simulink model "tmp_old"  (R2018b)
settings: Solver=VariableStepAuto  StartTime=0.0  StopTime=10.0  RelTol=1e-3
undefined symbols (not defined in the file or in its folder): GeRa, sigbuilder_block
libraries: fl_lib x63, sdl_lib x20, nesl_utility x11, simulink x7, dspswit3 x1
(part 1 of 3)
settings Model: Creator=Tanya  LastModifiedBy=Tanya

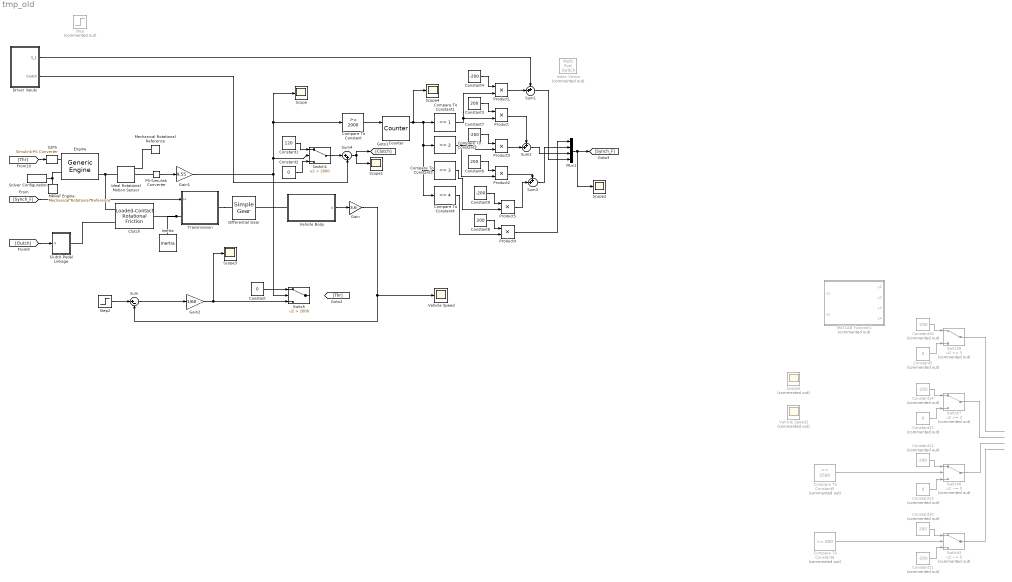
== system tmp_old ==
  Clutch : sdl_lib/Brakes & Detents/Rotational/Loaded-Contact Rotational Friction  geometry_model=1  r_eff=300 mm  d_o=150 mm  d_i=100 mm  friction_model=1  mu_coulomb=0.46  mu_w_vector=[ 0 0.1 0.2 0.3 0.4 0.5 1 2 5 10 100 1000 ] rad/s  mu_coulomb_vector=[ 0.29 0.28 0.26 0.22 0.21 0.2 0.2 0.19 0.19 0.19 0.19 0.19 ]  mu_interp_method=1  mu_extrap_method=1  mu_static=0.5  w_tol=0.001 rad/s  force_min=10 N  mu_visc=0 N*m/(rad/s)  initial_state_locked=0  temperature_TLU=[280.0, 300.0, 320.0] K  mu_coulomb_temp_vector=[0.3, 0.28, 0.25]  mu_coulomb_matrix=[0.34, 0.32, 0.3; 0.3, 0.28, 0.25; 0.25, 0.2, 0.15]  mu_static_vector=[0.4, 0.38, 0.36]  thermal_mass=50 kJ/K  T_init=300 K
      settings: SourceProductName=Simscape Driveline  SourceProductBaseCode=LD
  Clutch Pedal Linkage : Subsystem  Tag=PublishSubsystem
      mask Display:
      | color('white')
      | plot(-40,-80);
      | plot(40,40);
      | color('black'),
      | patch([-45 -30 -20 -20 -45],[-90 -90 -75 -55 -90]+20)
      | patch([-30 -10  5 10 20 [20 10 6 -10 -30]-2],[-55 -50 20 25 35 fliplr([-55 -50 20 25 35])-5]);
  Compare To Constant : simulink/Logic and Bit Operations/Compare To Constant  relop=>=  const=2000  OutDataTypeStr=boolean
  Compare To Constant1 : simulink/Logic and Bit Operations/Compare To Constant  relop===  const=1  OutDataTypeStr=uint8
  Compare To Constant2 : simulink/Logic and Bit Operations/Compare To Constant  relop===  const=2  OutDataTypeStr=uint8
  Compare To Constant3 : simulink/Logic and Bit Operations/Compare To Constant  relop===  const=3  OutDataTypeStr=uint8
  Compare To Constant4 : simulink/Logic and Bit Operations/Compare To Constant  relop===  const=4  OutDataTypeStr=uint8
  Compare To Constant5 : simulink/Logic and Bit Operations/Compare To Constant  Commented=on  relop=>=  const=2500  OutDataTypeStr=uint8
  Compare To Constant6 : simulink/Logic and Bit Operations/Compare To Constant  Commented=on  relop=>=  const=800  OutDataTypeStr=uint8
  Constant : Constant  Value=0
  Constant1 : Constant  Value=120
  Constant10 : Constant  Commented=on  Value=200
  Constant11 : Constant  Commented=on  Value=-200
  Constant12 : Constant  Commented=on  Value=200
  Constant13 : Constant  Commented=on  Value=0
  Constant14 : Constant  Commented=on  Value=-200
  Constant15 : Constant  Commented=on  Value=0
  Constant16 : Constant  Commented=on  Value=-200
  Constant2 : Constant  Value=0
  Constant3 : Constant  Value=200
  Constant4 : Constant  Value=-200
  Constant5 : Constant  Commented=on  Value=0
  Constant6 : Constant  Value=200
  Constant7 : Constant  Value=-200
  Constant8 : Constant  Value=200
  Constant9 : Constant  Value=-200
  Counter : dspswit3/Counter  Direction=Up  CountEvent=Rising edge  CounterSize=User defined  MaxCount=255  InitialCount=0  Output=Count and Hit  HitValue=32  ResetInput=on  SamplesPerFrame=1  Ts=1  CntDtype=double  HitDtype=Logical
  Differential Gear : sdl_lib/Gears/Simple Gear  ratio=4.3  rotation_direction=1  friction_model=2  T_noload=0.1 N*m  T_nom=5 N*m  efficiency_nom=0.8  efficiency=0.86  mu_visc=[0 0] N*m/(rad/s)  w_thr=0.01 rad/s  pwr_thr=0.001 W  enable_faults=0  efficiency_fault=0.05  external_fault=simscape.enum.onoff.off  temporal_fault=0  fault_time=5 s  fault_angles=pi / 12 rad  report_fault=1  temperature_TLU=[ 280 300 320 ] K  load_TLU=[ 1 5 10 ] N*m  efficiency_TLU=[ 0.95 0.9 0.85 ]  efficiency_TLU2=[ 0.85 0.8 0.75; 0.95 0.9 0.85; 0.85 0.8 0.7 ]  thermal_mass=50 J/K  T_init=300 K
      settings: SourceProductName=Simscape Driveline
  Driver inputs : Subsystem  Tag=STV Subsys  LoadFcn=sigbuilder_block('load');  StartFcn=sigbuilder_block('start');  StopFcn=sigbuilder_block('stop');  ClipboardFcn=sigbuilder_block('clipboard');  mask(Sigbuilder block){tuvar=[0:10]}
      mask help: Sigbuilder GUI
      mask init:
      | if ~strcmp(get_param(bdroot(gcbh),'SimulationStatus'),'stopped') tuvar = sigbuilder_block('maskInit'); end
      settings: CopyFcn=sigbuilder_block('copy');  DeleteFcn=sigbuilder_block('delete');  ModelCloseFcn=sigbuilder_block('modelClose');  PreSaveFcn=sigbuilder_block('preSave');  PauseFcn=sigbuilder_block('pause')  ContinueFcn=sigbuilder_block('continue')  NameChangeFcn=sigbuilder_block('namechange');  OpenFcn=sigbuilder_block('open',[187.8 152.4 619.2 435 ]);  CloseFcn=sigbuilder_block('close');
      mask Display: plot(0, 0, 100, 100,[2, 2, 32, 32, 2], [68, 8, 8, 68, 68],[32, 2], [38, 38], [32, 19, 2],[53, 60, 44], [32, 17, 17, 2],[16, 16, 31, 31]);txt = getActiveGroup(gcbh);text(2, 100, txt,'verticalAlignment', 'top');
  Engine : sdl_lib/Engines/Generic Engine  model_parameterization=1  engine_type=1  P_max=100e3 W  w_P_max=6500 rpm  w_max=8500 rpm  w_min=200 rpm  w_tab=[ 500 1000 2e+3 3e+3 4e+3 5e+3 6e+3 7e+3 ] rpm  trq_tab=[ 380 380 380 380 350 280 200 80 ] N*m  pwr_tab=[ 2e+4 4e+4 7.8e+4 1.2e+5 1.45e+5 1.48e+5 1.25e+5 6e+4 ] W  interp_method=simscape.enum.interpolation.linear  model_inertia=1  inertia=0.16 kg*m^2  initial_velocity=800 rpm  model_time_constant=1  time_constant=0.2 s  T0=0  w_thr=20 rpm  idle_speed=1  idle_speed_reference=800 rpm  tau_controller=.6 s  idle_w_thr=1 rpm  redline=0  redline_speed=5000 rpm  tau_redline=1 s  redline_w_thr=1 rpm  fc_model=0  fc_per_rev=25 mg/rev  displaced_volume=400 cm^3  rev_per_cycle=2  fc_w_tab=[ 1000 2e+3 3e+3 4e+3 5e+3 6e+3 ] rpm  fc_trq_tab=[ 0 80 160 200 240 320 360 400 ] N*m  fc_tab=[ 0.5 0.9 1.4 1.6 1.9 2.7 3.4 4.4; 1 1.7 2.7 3.1 3.6 5 6 7.4; 1.4 2.7 4 4.8 5.6 7.5 8.5 10.5; 2 3.6 5.8 6.7 8 10.4 11.7 13.3; 2.5 4.8 7.9 9.4 10.8 14 16.2 18.6; 3.1 6 10.3 11.9 13.8 18.4 22 26.5 ] g/s  bmep_tab=[ 0 250 500 625 750 1000 1.15e+3 1.25e+3 ] kPa  bsfc_tab=[ 410 380 300 280 270 290 320 380; 410 370 290 270 260 270 285 320; 415 380 290 275 265 270 270 300; 420 390 310 290 285 280 280 285; 430 410 340 320 310 300 310 320; 450 430 370 340 330 330 350 380 ] g/hr/kW  fc_interp_method=simscape.enum.interpolation.linear
      settings: SourceProductName=Simscape Driveline  SourceProductBaseCode=LD
  Gain : Gain  Gain=3.6
  Gain1 : Gain  Gain=9.55
  Gain2 : Gain  Gain=1/60
  Ideal Rotational Motion Sensor : fl_lib/Mechanical/Mechanical Sensors/Ideal Rotational Motion Sensor  offset=0 rad
  Index Vector : MultiPortSwitch  Commented=on  DataPortOrder=Zero-based contiguous  Inputs=2  zeroidx=on
  Inertia : fl_lib/Mechanical/Rotational Elements/Inertia  inertia=0.005 kg*m^2  w_specify=off  w_priority=High  w=0 rad/s  w_nominal_specify=off  w_nominal_unit=rad/s  w_nominal_value=1  t_specify=off  t_priority=High  t=0 N*m  t_nominal_specify=off  t_nominal_unit=N*m  t_nominal_value=1
  MATLAB Function1 : MATLAB Function  Commented=on  TreatAsAtomicUnit=on
  MRRef Engine : fl_lib/Mechanical/Rotational Elements/Mechanical Rotational Reference
  Mechanical Rotational Reference : fl_lib/Mechanical/Rotational Elements/Mechanical Rotational Reference
  Mux1 : Mux
  PS-Simulink Converter : nesl_utility/PS-Simulink Converter  PhysicalDomain=network_engine_domain  SubClassName=ps_output  LeftPortType=input  RightPortType=output  PseudoPeriodic=off  Frequencies=[]  Unit=rad/s  AffineConversion=off
  Product{,1..5} (6 alike) : Product
  S2PS : nesl_utility/Simulink-PS Converter  PhysicalDomain=network_engine_domain  SubClassName=ps_input  LeftPortType=input  RightPortType=output  PseudoPeriodic=off  Frequencies=[]  NoiseDistribution=none  NoiseParameters=[]  Unit=1  AffineConversion=off  FilteringAndDerivatives=zero  SimscapeFilterOrder=1  InputFilterTimeConstant=.001  UdotUserProvided=0
  Scope{,1..4} (5 alike) : Scope
  Scope5 : Scope  Commented=on
  Solver Configuration : nesl_utility/Solver Configuration  PhysicalDomain=network_engine_domain  SubClassName=solver  LeftPortType=input  RightPortType=generic  Tones=[]  Harmonics=[]  SimulateNoise=off  Profile=off  UseLocalSampling=off  EnableSwitchedLinearOptims=on  FrequencyDomain=off  UseCCode=off  RelTol=0.001  AbsTol=1e-06  MinStep=1e-09  ToWorkspace=off  RevertToSquareIcSolve=off  NumHomotopyIterations=100  PhasorMode=off  PhasorModeNumHarmonics=1  DoDC=off  ResidualTolerance=1e-9  UseLocalSolver=off  LocalSolverChoice=NE_BACKWARD_EULER_ADVANCER  LocalSolverSampleTime=.001  DoFixedCost=off  MaxNonlinIter=3  MaxModeIter=2  LinearAlgebra=auto  EquationFormulation=NE_TIME_EF  DelaysMemoryBudget=1024  AutomaticFiltering=on  FilteringTimeConstant=0.001  PartitionStorageMethod=AS_NEEDED  PartitionMemoryBudget=1024
  Step : Step  Commented=on  Time=3.6  After=0.1  SampleTime=0
  Step2 : Step  Time=3.6  After=60  SampleTime=0
  Sum : Sum  Inputs=|+-
  Sum1 : Sum  Inputs=++|
  Sum2 : Sum  Inputs=++|
  Sum3 : Sum  Inputs=++|
  Sum4 : Sum  Inputs=|++
  Switch : Switch  Criteria=u2 > Threshold  Threshold=2000
  Switch1 : Switch  Criteria=u2 > Threshold  Threshold=2000
  Switch2 : Switch  Commented=on  Criteria=u2 ~= 0  Threshold=2000
  Switch6 : Switch  Commented=on  Criteria=u2 ~= 0  Threshold=1.6
  Switch7 : Switch  Commented=on  Threshold=2
  Switch8 : Switch  Commented=on  Threshold=3
  Transmission : Subsystem  VariantControlMode=Label  Variant=on  LabelModeActiveChoice=Detailed
      settings: AttributesFormatString=%<ActiveVariant>
      mask Display:
      | blk = find_system(gcbh, 'SearchDepth', 1, 'Parent', gcb, 'VariantObject', get_param(gcb,'activevariant'));
      | eval(get_param(blk, 'MaskDisplay'));
  Vehicle Speed : Scope
  Vehicle Speed1 : Scope  Commented=on
  Vehicle Body : Subsystem  Tag=PublishSubsystem
      mask Display:
      | color('white')
      | plot(-120,-60); plot(120,50);
      | color('black')
      | plot(sin(0:0.1:6*pi)*15-70,cos(0:0.1:6*pi)*15-30);
      | plot(sin(0:0.1:6*pi)*15+70,cos(0:0.1:6*pi)*15-30);
      | plot([-88 -95 -99 -99 -95 -75 -65 -50 -46 10 30 34 80 85 90 93 95 93 90 88],[-30 -28 -23 -5 0 5 10 20 21 21 0 -2 -7 -9 -13 -17 -25 -28 -30 -30])
      | plot([-88 -95 -99 -99 -95 -75 -65 -50 -46 10 30 34 80 85 90 93 95 93 90 88],[-30 -28 -23 -5 0 5 10 20 21 21 0 -2 -7 -9 -13 -17 -25 -28 -30 -30]-1)
      | plot([-88 -95 -99 -99 -95 -75 -65 -50 -46 10 30 34 80 85 90 93 95 93 90 88]+1,[-30 -28 -23 -5 0 5 10 20 21 21 0 -2 -7 -9 -13 -17 -25 -28 -30 -30])
      | plot([-50 50],[-30 -30])
  wires:
  Driver inputs/1(S_1) -> Sum1/1
  Constant6/1 -> Product2/1
  Product2/1 -> Sum3/1
  Constant4/1 -> Product1/1
  Product3/1 -> Sum2/2
  Counter/1 -> Scope4/1, Compare To Constant4/1, Compare To Constant3/1, Compare To Constant2/1, Compare To Constant1/1
  Compare To Constant3/1 -> Product5/2
  Product5/1 -> Sum3/2
  [Clutch] -> Clutch Pedal Linkage/1(S)
  Step2/1 -> Sum/1
  [Synch_F] -> Transmission/1(H)
  Compare To Constant/1 -> Counter/1
  Constant7/1 -> Product3/1
  Product4/1 -> Mux1/1
  Compare To Constant4/1 -> Product4/2
  Vehicle Body/1(V) -> Gain/1
  Constant8/1 -> Product4/1
  Constant9/1 -> Product5/1
  Compare To Constant1/1 -> Product1/2, Product/2
  Product/1 -> Sum2/1
  Mux1/1 -> [Synch_F], Scope2/1
  Constant2/1 -> Switch1/3
  PS-Simulink Converter/1 -> Gain1/1
  Gain2/1 -> Scope3/1, Switch/3
  Sum2/1 -> Mux1/3
  Sum4/1 -> [Clutch], Scope1/1
  Product1/1 -> Sum1/2
  Sum3/1 -> Mux1/2
  Compare To Constant2/1 -> Product2/2, Product3/2
  Constant/1 -> Switch/1
  Switch1/1 -> Sum4/1
  Sum/1 -> Gain2/1
  Constant3/1 -> Product/1
  Driver inputs/2(Clutch) -> Sum4/2
  [Thr] -> S2PS/1
  Sum1/1 -> Mux1/4
  Constant1/1 -> Switch1/1
  Gain1/1 -> Scope/1, Compare To Constant/1, Switch1/2, Switch/2
  Gain/1 -> Sum/2, Vehicle Speed/1
  Switch7/1 -> ?
  ? -> MATLAB Function1/1(u1), Switch8/2, Switch7/2, Compare To Constant5/1, Compare To Constant6/1, Scope5/1
  Constant16/1 -> Switch8/1
  Compare To Constant6/1 -> Switch2/2
  Constant5/1 -> Switch8/3
  Switch8/1 -> ?
  Compare To Constant5/1 -> Switch6/2
  Constant10/1 -> Switch2/1
  Constant14/1 -> Switch7/1
  Constant12/1 -> Switch6/1
  Switch6/1 -> ?
  ? -> Vehicle Speed1/1
  Switch2/1 -> ?
  Constant13/1 -> Switch6/3
  Constant11/1 -> Switch2/3
  Constant15/1 -> Switch7/3
  connections:
  MRRef Engine/LConn1 -- Solver Configuration/RConn1 -- Engine/LConn2
  Transmission/LConn1 -- Clutch/RConn1 -- Inertia/LConn1
  Ideal Rotational Motion Sensor/LConn1 -- Clutch/LConn2 -- Engine/RConn3
  Mechanical Rotational Reference/LConn1 -- Ideal Rotational Motion Sensor/RConn1
  Engine/LConn1 -- S2PS/RConn1
  Clutch/LConn1 -- Clutch Pedal Linkage/RConn1
  Transmission/RConn1 -- Differential Gear/LConn1
  PS-Simulink Converter/LConn1 -- Ideal Rotational Motion Sensor/RConn2
  Vehicle Body/LConn1 -- Differential Gear/RConn1

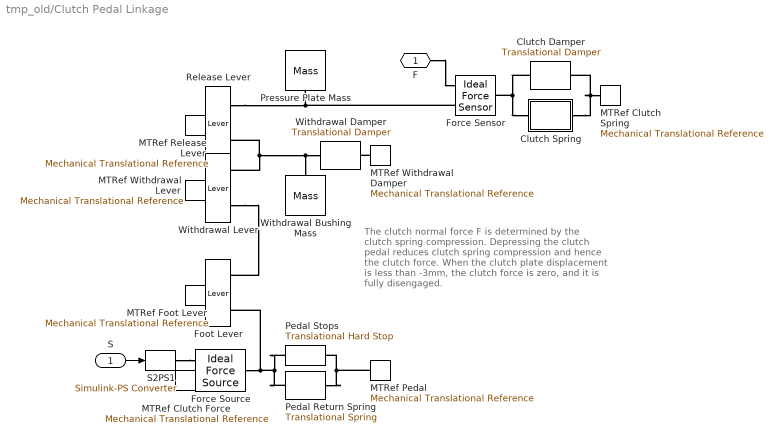
== system tmp_old/Clutch Pedal Linkage ==
  note: The clutch normal force F is determined by the
      | clutch spring compression. Depressing the
      | clutch pedal reduces clutch spring compression
      | and hence the clutch force. When the clutch plate
      | displacement is less than -3mm, the
      | clutch force is zero, and it is fully disengaged.
  S : Inport
  Clutch Damper : fl_lib/Mechanical/Translational Elements/Translational Damper  D=100 N/(m/s)  v_specify=off  v_priority=High  v=0 m/s  v_nominal_specify=off  v_nominal_unit=m/s  v_nominal_value=1  f_specify=off  f_priority=High  f=0 N  f_nominal_specify=off  f_nominal_unit=N  f_nominal_value=1
  Clutch Spring : Subsystem
  Foot Lever : fl_lib/Mechanical/Mechanisms/Lever  arm_AC=76 mm  arm_BC=148 mm  f_A_specify=off  f_A_priority=High  f_A=0 N  f_A_nominal_specify=off  f_A_nominal_unit=N  f_A_nominal_value=1  f_B_specify=off  f_B_priority=High  f_B=0 N  f_B_nominal_specify=off  f_B_nominal_unit=N  f_B_nominal_value=1  f_C_specify=off  f_C_priority=High  f_C=0 N  f_C_nominal_specify=off  f_C_nominal_unit=N  f_C_nominal_value=1
      settings: SourceProductName=Simscape  SourceProductBaseCode=SS
  Force Sensor : fl_lib/Mechanical/Mechanical Sensors/Ideal Force Sensor
  Force Source : fl_lib/Mechanical/Mechanical Sources/Ideal Force Source
  MTRef Clutch Force : fl_lib/Mechanical/Translational Elements/Mechanical Translational Reference
  MTRef Foot Lever : fl_lib/Mechanical/Translational Elements/Mechanical Translational Reference
  MTRef Release Lever : fl_lib/Mechanical/Translational Elements/Mechanical Translational Reference
  MTRef Withdrawal Damper : fl_lib/Mechanical/Translational Elements/Mechanical Translational Reference
  MTRef Withdrawal Lever : fl_lib/Mechanical/Translational Elements/Mechanical Translational Reference
  "MTRef Clutch Spring " : fl_lib/Mechanical/Translational Elements/Mechanical Translational Reference
  MTRef Pedal : fl_lib/Mechanical/Translational Elements/Mechanical Translational Reference
  Pedal Return Spring : fl_lib/Mechanical/Translational Elements/Translational Spring  spr_rate=120 N/m  v_specify=off  v_priority=High  v=0 m/s  v_nominal_specify=off  v_nominal_unit=m/s  v_nominal_value=1  f_specify=off  f_priority=High  f=0 N  f_nominal_specify=off  f_nominal_unit=N  f_nominal_value=1  x_specify=on  x_priority=High  x=1.5 cm  x_nominal_specify=off  x_nominal_unit=m  x_nominal_value=1
  Pedal Stops : fl_lib/Mechanical/Translational Elements/Translational Hard Stop  upper_bnd=168 mm  lower_bnd=0 mm  stiff_up=1e6 N/m  stiff_low=1e6 N/m  D_up=150 N/(m/s)  D_low=150 N/(m/s)  model=3  transition=0.1 mm  v_specify=off  v_priority=High  v=0 m/s  v_nominal_specify=off  v_nominal_unit=m/s  v_nominal_value=1  f_specify=off  f_priority=High  f=0 N  f_nominal_specify=off  f_nominal_unit=N  f_nominal_value=1  x_specify=off  x_priority=High  x=0 m  x_nominal_specify=off  x_nominal_unit=m  x_nominal_value=1
  Pressure Plate Mass : fl_lib/Mechanical/Translational Elements/Mass  mass=4.2 kg  v_specify=off  v_priority=High  v=0 m/s  v_nominal_specify=off  v_nominal_unit=m/s  v_nominal_value=1  f_specify=off  f_priority=High  f=0 N  f_nominal_specify=off  f_nominal_unit=N  f_nominal_value=1
  Release Lever : fl_lib/Mechanical/Mechanisms/Lever  arm_AC=7.2 mm  arm_BC=38 mm  f_A_specify=off  f_A_priority=High  f_A=0 N  f_A_nominal_specify=off  f_A_nominal_unit=N  f_A_nominal_value=1  f_B_specify=off  f_B_priority=High  f_B=0 N  f_B_nominal_specify=off  f_B_nominal_unit=N  f_B_nominal_value=1  f_C_specify=off  f_C_priority=High  f_C=0 N  f_C_nominal_specify=off  f_C_nominal_unit=N  f_C_nominal_value=1
      settings: SourceProductName=Simscape  SourceProductBaseCode=SS
  S2PS1 : nesl_utility/Simulink-PS Converter  PhysicalDomain=network_engine_domain  SubClassName=ps_input  LeftPortType=input  RightPortType=output  PseudoPeriodic=off  Frequencies=[]  NoiseDistribution=none  NoiseParameters=[]  Unit=1  AffineConversion=off  FilteringAndDerivatives=filter  SimscapeFilterOrder=1  InputFilterTimeConstant=.001  UdotUserProvided=0
  Withdrawal Bushing Mass : fl_lib/Mechanical/Translational Elements/Mass  mass=0.6 kg  v_specify=off  v_priority=High  v=0 m/s  v_nominal_specify=off  v_nominal_unit=m/s  v_nominal_value=1  f_specify=off  f_priority=High  f=0 N  f_nominal_specify=off  f_nominal_unit=N  f_nominal_value=1
  Withdrawal Lever : fl_lib/Mechanical/Mechanisms/Lever  arm_AC=42 mm  arm_BC=128 mm  f_A_specify=off  f_A_priority=High  f_A=0 N  f_A_nominal_specify=off  f_A_nominal_unit=N  f_A_nominal_value=1  f_B_specify=off  f_B_priority=High  f_B=0 N  f_B_nominal_specify=off  f_B_nominal_unit=N  f_B_nominal_value=1  f_C_specify=off  f_C_priority=High  f_C=0 N  f_C_nominal_specify=off  f_C_nominal_unit=N  f_C_nominal_value=1
      settings: SourceProductName=Simscape  SourceProductBaseCode=SS
  Withdrawal Damper : fl_lib/Mechanical/Translational Elements/Translational Damper  D=100 N/(m/s)  v_specify=off  v_priority=High  v=0 m/s  v_nominal_specify=off  v_nominal_unit=m/s  v_nominal_value=1  f_specify=off  f_priority=High  f=0 N  f_nominal_specify=off  f_nominal_unit=N  f_nominal_value=1
  F : PMIOPort  Side=Right
  wires:
  S/1 -> S2PS1/1
  connections:
  MTRef Foot Lever/LConn1 -- Foot Lever/RConn1
  MTRef Pedal/LConn1 -- Pedal Return Spring/RConn1 -- Pedal Stops/RConn1
  MTRef Withdrawal Damper/LConn1 -- Withdrawal Damper/RConn1
  MTRef Release Lever/LConn1 -- Release Lever/RConn1
  Withdrawal Lever/LConn2 -- Foot Lever/LConn1
  MTRef Withdrawal Lever/LConn1 -- Withdrawal Lever/RConn1
  Withdrawal Lever/LConn1 -- Release Lever/LConn2 -- Withdrawal Bushing Mass/LConn1 -- Withdrawal Damper/LConn1
  Release Lever/LConn1 -- Force Sensor/RConn1 -- Pressure Plate Mass/LConn1
  Pedal Stops/LConn1 -- Pedal Return Spring/LConn1 -- Force Source/LConn1 -- Foot Lever/LConn2
  "MTRef Clutch Spring "/LConn1 -- Clutch Spring/RConn1 -- Clutch Damper/RConn1
  Clutch Spring/LConn1 -- Clutch Damper/LConn1 -- Force Sensor/LConn1
  F/RConn1 -- Force Sensor/RConn2
  MTRef Clutch Force/LConn1 -- Force Source/RConn2
  S2PS1/RConn1 -- Force Source/RConn1

== system tmp_old/Driver inputs ==
  Demux : Demux  Tag=STV Demux  Outputs=2
  FromWs : FromWorkspace  Tag=STV FromWs  VariableName=tuvar  SampleTime=0
      SigBuilderData=|
      | common.afterFinalStr = 'Extrapolate'
      | common.sampleTime = 0
      | dataSet.timeRange = [0 30]
      | dataSet.name = 'Group 1'
      | sbobj.Groups.Name = 'Group 1'
      | sbobj.Groups.Signals(1).Name = 'S_1'
      | sbobj.Groups.Signals(1).XData = [0 1.7 1.85 3.25 3.35 8.35 8.5 9.3 9.3 9.4 30]
      | sbobj.Groups.Signals(1).YData = [0 0 200 200 0 0 0 -2 0 0 0]
      | sbobj.Groups.Signals(2).Name = 'Clutch'
      | sbobj.Groups.Signals(2).XData = [0 0.95 1.45 3.5 4 8.15 8.35 8.35 10 10.4 15.4 15.8 17.2 17.7 22.5 22.8 24.3 24.6 30]
      | sbobj.Groups.Signals(2).YData = [0 0 120 120 0 0 1 0 0 0 0 0 0 0 0 0 0 0 0]
      | sbobj.Groups.TimeRange = [0 30]
  S_1 : Outport  Tag=STV Outport
  Clutch : Outport  Tag=STV Outport  Port=2
  wires:
  FromWs/1 -> Demux/1
  Demux/1 -> S_1/1
  Demux/2 -> Clutch/1

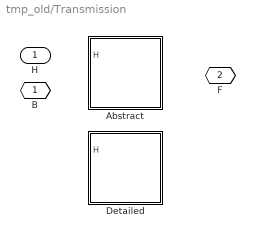
== system tmp_old/Transmission ==
  H : Inport
  Abstract : Subsystem  Tag=PublishSubsystem  VariantControl=Abstract
      mask Display:
      | patch([-20;320.146012604237;320.146012604237;-20;-20], [340.146012604237;340.146012604237;0;0;340.146012604237],[1 1 1])
      | plot([195.583957247436;209.756707772613], [274.951360188425;260.778609663248])
      | plot([209.756707772613;195.583957247436], [274.951360188425;260.778609663248])
      | plot([184.245756827295;198.418507352471], [76.5328528359532;62.3601023107767])
      | plot([198.418507352471;184.245756827295], [76.5328528359532;62.3601023107767])
      | plot([99.2092536762357;99.2092536762357;141.727505251765;141.727505251765;99.2092536762357], [325.97326207906;212.591257877648;255.109509453177;283.455010503531;325.97326207906])
      | patch([136.058405041695;184.245756827295;198.418507352471;121.885654516518;136.058405041695], [289.124110713601;289.124110713601;303.296861238778;303.296861238778;289.124110713601], [0;0;0])
      | plot([136.058405041695;184.245756827295;198.418507352471;121.885654516518;136.058405041695], [289.124110713601;289.124110713601;303.296861238778;303.296861238778;289.124110713601])
      | patch([141.727505251765;141.727505251765;178.576656617224;178.576656617224;141.727505251765], [274.951360188425;266.447709873319;266.447709873319;274.951360188425;274.951360188425], [0;0;0])
      | plot([141.727505251765;141.727505251765;178.576656617224;178.576656617224;141.727505251765], [274.951360188425;266.447709873319;266.447709873319;274.951360188425;274.951360188425])
      | plot([221.094908192754;221.094908192754;178.576656617224;178.576656617224;221.094908192754], [325.97326207906;212.591257877648;255.109509453177;283.455010503531;325.97326207906])
      | patch([70.8637526258826;70.8637526258826;99.2092536762357;99.2092536762357;70.8637526258826], [272.116810083389;263.613159768283;263.613159768283;272.116810083389;272.116810083389], [0;0;0])
      | plot([70.8637526258826;70.8637526258826;99.2092536762357;99.2092536762357;70.8637526258826], [272.116810083389;263.613159768283;263.613159768283;272.116810083389;272.116810083389])
      | patch([221.094908192754;221.094908192754;249.440409243107;249.440409243107;221.094908192754], [272.116810083389;263.613159768283;263.613159768283;272.116810083389;272.116810083389], [0;0;0])
      | plot([221.094908192754;221.094908192754;249.440409243107;249.440409243107;221.094908192754], [272.116810083389;263.613159768283;263.613159768283;272.116810083389;272.116810083389])
      | plot([198.418507352471;198.418507352471], [235.26765871793;119.051104411483])
      | plot([121.885654516518;121.885654516518], [235.26765871793;119.051104411483])
      | plot([113.382004201412;113.382004201412;155.900255776942;155.900255776942;113.382004201412], [127.554754726589;14.1727505251765;56.6910021007061;85.0365031510592;127.554754726589])
      | patch([136.058405041695;184.245756827295;198.418507352471;121.885654516518;136.058405041695], [36.849151365459;36.849151365459;22.6764008402824;22.6764008402824;36.849151365459], [0;0;0])
      | plot([136.058405041695;184.245756827295;198.418507352471;121.885654516518;136.058405041695], [36.849151365459;36.849151365459;22.6764008402824;22.6764008402824;36.849151365459])
      | patch([85.0365031510592;85.0365031510592;113.382004201412;113.382004201412;85.0365031510592], [73.6983027309179;65.194652415812;65.194652415812;73.6983027309179;73.6983027309179], [0;0;0])
      | plot([85.0365031510592;85.0365031510592;113.382004201412;113.382004201412;85.0365031510592], [73.6983027309179;65.194652415812;65.194652415812;73.6983027309179;73.6983027309179])
      | plot([206.922157667577;206.922157667577;164.403906092048;164.403906092048;206.922157667577], [127.554754726589;14.1727505251765;56.6910021007061;85.0365031510592;127.554754726589])
      | patch([206.922157667577;206.922157667577;246.605859138072;246.605859138072;206.922157667577], [73.6983027309179;65.194652415812;65.194652415812;73.6983027309179;73.6983027309179], [0;0;0])
      | plot([206.922157667577;206.922157667577;246.605859138072;246.605859138072;206.922157667577], [73.6983027309179;65.194652415812;65.194652415812;73.6983027309179;73.6983027309179])
      | patch([155.900255776942;155.900255776942;164.403906092048;164.403906092048;155.900255776942], [76.5328528359532;68.0292025208473;68.0292025208473;76.5328528359532;76.5328528359532], [0;0;0])
      | plot([155.900255776942;155.900255776942;164.403906092048;164.403906092048;155.900255776942], [76.5328528359532;68.0292025208473;68.0292025208473;76.5328528359532;76.5328528359532])
  Detailed : Subsystem  Tag=PublishSubsystem  VariantControl=Detailed
      mask Display:
      | plot([225.488460855559;225.439323974897;225.292386547934;225.049063662416;224.711698650743;224.283540522401;223.76871267422;223.172173179813;222.499667040612;221.757670858367;220.953330461928;220.094392089012;219.189127785692;218.246255742078;217.274856331375;216.28428466093;215.284080477431;214.283876293932;213.293304623488;212.321905212785;211.379033169171;210.473768865851;209.614830492935;208.810490096496;208.068493914251;207.39598777505;206.799448280642;206.284620432462;205.85646230412;205.519097292447;205.275774406929;205.128836979966;205.079700099304;205.128836979966;205.275774406929;205.519097292447;205.85646230412;206.284620432462;206.799448280642;207.39598777505;208.068493914251;208.810490096496;209.614830492935;210.473768865851;211.379033169171;212.321905212785;213.293304623488;214.283876293932;215.284080477431;216.28428466093;217.274856331375;218.246255742078;219.189127785692;220.094392089012;220.953330461928;221.757670858367;222.499667040612;223.172173179813;223.76871267422;224.283540522401;224.711698650743;225.049063662416;225.292386547934;225.439323974897;225.488460855559;225.488460855559], [194.182429695502;193.182225512003;192.191653841558;191.220254430856;190.277382387241;189.372118083922;188.513179711005;187.708839314567;186.966843132321;186.29433699312;185.697797498713;185.182969650533;184.75481152219;184.417446510518;184.174123624999;184.027186198036;183.978049317375;184.027186198036;184.174123624999;184.417446510518;184.75481152219;185.182969650533;185.697797498713;186.29433699312;186.966843132321;187.708839314567;188.513179711005;189.372118083922;190.277382387241;191.220254430856;192.191653841558;193.182225512003;194.182429695502;195.182633879001;196.173205549446;197.144604960148;198.087477003763;198.992741307082;199.851679679999;200.656020076437;201.398016258683;202.070522397884;202.667061892291;203.181889740471;203.610047868813;203.947412880486;204.190735766005;204.337673192967;204.386810073629;204.337673192967;204.190735766005;203.947412880486;203.610047868813;203.181889740471;202.667061892291;202.070522397884;201.398016258683;200.656020076437;199.851679679999;198.992741307082;198.087477003763;197.144604960148;196.173205549446;195.182633879001;194.182429695502;194.182429695502])
      | plot([225.488460855559;225.439323974897;225.292386547934;225.049063662416;224.711698650743;224.283540522401;223.76871267422;223.172173179813;222.499667040612;221.757670858367;220.953330461928;220.094392089012;219.189127785692;218.246255742078;217.274856331375;216.28428466093;215.284080477431;214.283876293932;213.293304623488;212.321905212785;211.379033169171;210.473768865851;209.614830492935;208.810490096496;208.068493914251;207.39598777505;206.799448280642;206.284620432462;205.85646230412;205.519097292447;205.275774406929;205.128836979966;205.079700099304;205.128836979966;205.275774406929;205.519097292447;205.85646230412;206.284620432462;206.799448280642;207.39598777505;208.068493914251;208.810490096496;209.614830492935;210.473768865851;211.379033169171;212.321905212785;213.293304623488;214.283876293932;215.284080477431;216.28428466093;217.274856331375;218.246255742078;219.189127785692;220.094392089012;220.953330461928;221.757670858367;222.499667040612;223.172173179813;223.76871267422;224.283540522401;224.711698650743;225.049063662416;225.292386547934;225.439323974897;225.488460855559;225.488460855559], [155.002648243681;154.002444060182;153.011872389737;152.040472979034;151.09760093542;150.1923366321;149.333398259184;148.529057862746;147.7870616805;147.114555541299;146.518016046892;146.003188198711;145.575030070369;145.237665058697;144.994342173178;144.847404746215;144.798267865553;144.847404746215;144.994342173178;145.237665058697;145.575030070369;146.003188198711;146.518016046892;147.114555541299;147.7870616805;148.529057862746;149.333398259184;150.1923366321;151.09760093542;152.040472979034;153.011872389737;154.002444060182;155.002648243681;156.00285242718;156.993424097624;157.964823508327;158.907695551941;159.812959855261;160.671898228177;161.476238624616;162.218234806861;162.890740946062;163.48728044047;164.00210828865;164.430266416992;164.767631428665;165.010954314183;165.157891741146;165.207028621808;165.157891741146;165.010954314183;164.767631428665;164.430266416992;164.00210828865;163.48728044047;162.890740946062;162.218234806861;161.476238624616;160.671898228177;159.812959855261;158.907695551941;157.964823508327;156.993424097625;156.00285242718;155.002648243681;155.002648243681])
      | plot([137.995347613469;137.946210732807;137.799273305844;137.555950420326;137.218585408653;136.790427280311;136.275599432131;135.679059937724;135.006553798522;134.264557616277;133.460217219838;132.601278846922;131.696014543602;130.753142499988;129.781743089286;128.791171418841;127.790967235342;126.790763051843;125.800191381398;124.828791970695;123.885919927081;122.980655623761;122.121717250845;121.317376854407;120.575380672161;119.90287453296;119.306335038553;118.791507190372;118.36334906203;118.025984050358;117.782661164839;117.635723737876;117.586586857215;117.635723737876;117.782661164839;118.025984050358;118.36334906203;118.791507190372;119.306335038553;119.90287453296;120.575380672161;121.317376854407;122.121717250845;122.980655623761;123.885919927081;124.828791970695;125.800191381398;126.790763051843;127.790967235342;128.791171418841;129.781743089286;130.753142499988;131.696014543602;132.601278846922;133.460217219838;134.264557616277;135.006553798522;135.679059937723;136.275599432131;136.790427280311;137.218585408653;137.555950420326;137.799273305844;137.946210732807;137.995347613469;137.995347613469], [275.187572697178;274.187368513678;273.196796843234;272.225397432531;271.282525388917;270.377261085597;269.518322712681;268.713982316242;267.971986133997;267.299479994796;266.702940500388;266.188112652208;265.759954523866;265.422589512193;265.179266626675;265.032329199712;264.98319231905;265.032329199712;265.179266626675;265.422589512193;265.759954523866;266.188112652208;266.702940500389;267.299479994796;267.971986133997;268.713982316242;269.518322712681;270.377261085597;271.282525388917;272.225397432531;273.196796843234;274.187368513678;275.187572697178;276.187776880677;277.178348551121;278.149747961824;279.092620005438;279.997884308758;280.856822681674;281.661163078113;282.403159260358;283.075665399559;283.672204893967;284.187032742147;284.615190870489;284.952555882162;285.19587876768;285.342816194643;285.391953075305;285.342816194643;285.19587876768;284.952555882162;284.615190870489;284.187032742147;283.672204893967;283.075665399559;282.403159260358;281.661163078113;280.856822681674;279.997884308758;279.092620005438;278.149747961824;277.178348551121;276.187776880677;275.187572697178;275.187572697178])
      | plot([99.4454661849886;116.4527668152;116.4527668152;139.129167655483;139.129167655483;198.654719861224;156.136468285695;156.136468285695;195.820169756189;99.4454661849886;99.4454661849886], [272.353022592142;272.353022592142;241.172971436754;241.172971436754;272.353022592142;272.353022592142;229.834771016613;116.4527668152;73.9345152396709;73.9345152396709;272.353022592142])
      | plot([113.618216710165;127.790967235342;141.963717760518;190.151069546118;190.151069546118;161.805568495765;161.805568495765], [278.022122802213;295.029423432425;278.022122802213;278.022122802213;303.533073747531;303.533073747531;278.022122802213])
      | plot([113.618216710165;127.790967235342;141.963717760518;190.151069546118;190.151069546118;161.805568495765;161.805568495765], [68.2654150296003;51.2581143993884;68.2654150296003;68.2654150296003;42.7544640842825;42.7544640842825;68.2654150296003])
      | plot([161.805568495765;190.151069546118], [303.533073747531;278.022122802213])
      | plot([161.805568495765;190.151069546118], [278.022122802213;303.533073747531])
      | plot([161.805568495765;190.151069546118], [68.2654150296003;42.7544640842825])
      | plot([161.805568495765;190.151069546118], [42.7544640842825;68.2654150296003])
      | plot([241.172971436754;278.022122802213], [272.353022592142;272.353022592142])
      | plot([241.172971436754;278.022122802213], [73.9345152396709;73.9345152396709])
      | plot([241.172971436754;278.022122802213], [272.353022592142;303.533073747531])
      | plot([241.172971436754;278.022122802213], [303.533073747531;272.353022592142])
      | plot([241.172971436754;278.022122802213], [73.9345152396709;42.7544640842825])
      | plot([241.172971436754;278.022122802213], [42.7544640842825;73.9345152396709])
      | plot([184.481969336048;227.000220911577;241.172971436754;241.172971436754;278.022122802213;278.022122802213;278.022122802213;241.172971436754;241.172971436754;227.000220911577;184.481969336048;184.481969336048], [229.834771016613;272.353022592142;272.353022592142;303.533073747531;303.533073747531;244.007521541789;42.7544640842825;42.7544640842825;73.9345152396709;73.9345152396709;116.4527668152;229.834771016613])
      | plot([184.481969336048;249.67662175186;249.67662175186;184.481969336048], [215.662020491436;215.662020491436;130.625517340377;130.625517340377])
      | plot([207.15837017633;224.165670806542], [207.15837017633;207.15837017633])
      | plot([207.15837017633;224.165670806542], [141.963717760518;141.963717760518])
      | %plot([71.0999651346356;227.000220911577], [173.143768915907;173.143768915907])
      | plot([136.294617550448;116.4527668152;136.294617550448;119.287316920236;136.294617550448;119.287316920236;136.294617550448;119.287316920236], [269.518472487107;269.518472487107;261.014822172001;258.180272066966;252.511171856895;249.67662175186;246.842071646824;241.172971436754])
      | %plot([0.236212508752942;71.0999651346356;71.0999651346356], [258.180272066966;258.180272066966;278.022122802213])
      | %plot([0.236212508752942;71.0999651346356;71.0999651346356], [88.1072657648474;88.1072657648474;173.143768915907])
      | patch([0;357.625738251954;357.625738251954;0;0;0.472425017505884;0.472425017505884;357.153313234448;357.153313234448;0.472425017505884;0], [343.452987726778;343.452987726778;0;0;343.452987726778;342.980562709272;0.472425017505884;0.472425017505884;342.980562709272;342.980562709272;343.452987726778], [1;1;1])
      | plot([99.4454661849886;113.618216710165], [244.007521541789;258.180272066966])
      | plot([99.4454661849886;124.956417130306], [215.662020491436;241.172971436754])
      | plot([99.4454661849886;184.481969336048], [187.316519441083;272.353022592142])
      | plot([139.129167655483;156.136468285695], [255.34572196193;272.353022592142])
      | plot([99.4454661849886;156.136468285695], [158.97101839073;215.662020491436])
      | plot([99.4454661849886;156.136468285695], [130.625517340377;187.316519441083])
      | plot([99.4454661849886;156.136468285695], [102.280016290024;158.97101839073])
      | plot([99.4454661849886;156.136468285695], [73.9345152396709;130.625517340377])
      | plot([127.790967235342;161.805568495765], [73.9345152396709;110.78366660513])
      | plot([156.136468285695;175.978319020942], [73.9345152396709;93.776365974918])
      | plot([255.34572196193;278.022122802213], [272.353022592142;249.67662175186])
      | plot([227.000220911577;278.022122802213], [272.353022592142;221.331120701507])
      | plot([212.827470386401;278.022122802213], [258.180272066966;192.985619651154])
      | plot([198.654719861224;227.000220911577], [244.007521541789;215.662020491436])
      | plot([249.67662175186;278.022122802213], [192.985619651154;164.640118600801])
      | plot([198.654719861224;184.481969336048], [215.662020491436;229.834771016613])
      | plot([249.67662175186;278.022122802213], [164.640118600801;136.294617550448])
      | plot([249.67662175186;278.022122802213], [139.129167655483;110.78366660513])
      | plot([278.022122802213;227.000220911577], [79.6036154497415;130.625517340377])
      | plot([198.654719861224;255.34572196193], [130.625517340377;73.9345152396709])
  B : PMIOPort  Side=Left
  F : PMIOPort  Port=2  Side=Right

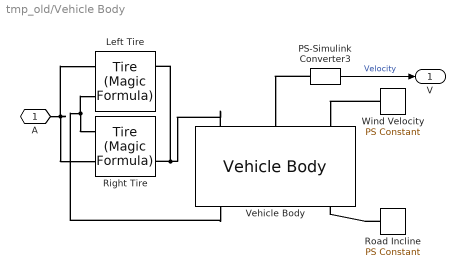
== system tmp_old/Vehicle Body ==
  Left Tire : sdl_lib/Tires & Vehicles/Tire (Magic Formula)  parameterization=3  F_z1=3000 N  F_x1=3500 N  kappa1=10  B_m=10  C_m=1.9  D_m=1  E_m=0.97  fz0=4e+3 N  p_Cx=1.685  p_Dx=[ 1.21 -0.037 ]  p_Ex=[ 0.344 0.095 -0.02 0 ]  p_Kx=[ 21.51 -0.163 0.245 ]  p_Hx=[ -0.002 0.002 ]  p_Vx=[ 0 0 ]  v_tr_thr=0.1 m/s  r_e=0.329 m  model_compliance=0  stiffness=1e+6 N/m  damping=1000 N/(m/s)  model_inertia=1  inertia=0.8 kg*m^2  initial_velocity=0 rpm  model_resistance=0  resistance_model=1  coeff=0.015  p_tire=250e3 Pa  alpha=-0.003  beta=0.97  coeff_a=84e-4  coeff_b=6.2e-4 s/m  coeff_c=1.6e-4 s^2/m^2  v_thr=1e-3 m/s
      settings: SourceProductName=Simscape Driveline
  PS-Simulink Converter3 : nesl_utility/PS-Simulink Converter  PhysicalDomain=network_engine_domain  SubClassName=ps_output  LeftPortType=input  RightPortType=output  PseudoPeriodic=off  Frequencies=[]  Unit=m/s  AffineConversion=off
  Right Tire : sdl_lib/Tires & Vehicles/Tire (Magic Formula)  parameterization=3  F_z1=3000 N  F_x1=3500 N  kappa1=10  B_m=10  C_m=1.9  D_m=1  E_m=0.97  fz0=4e+3 N  p_Cx=1.685  p_Dx=[ 1.21 -0.037 ]  p_Ex=[ 0.344 0.095 -0.02 0 ]  p_Kx=[ 21.51 -0.163 0.245 ]  p_Hx=[ -0.002 0.002 ]  p_Vx=[ 0 0 ]  v_tr_thr=0.1 m/s  r_e=0.329 m  model_compliance=0  stiffness=1e+6 N/m  damping=1000 N/(m/s)  model_inertia=1  inertia=0.8 kg*m^2  initial_velocity=0 rpm  model_resistance=0  resistance_model=1  coeff=0.015  p_tire=250e3 Pa  alpha=-0.003  beta=0.97  coeff_a=84e-4  coeff_b=6.2e-4 s/m  coeff_c=1.6e-4 s^2/m^2  v_thr=1e-3 m/s
      settings: SourceProductName=Simscape Driveline
  Road Incline : fl_lib/Physical Signals/Sources/PS Constant  constant=0
  Vehicle Body : sdl_lib/Tires & Vehicles/Vehicle Body  mass=3500 kg  n_w=2  x_f=1.4 m  x_r=1.6 m  y_c=1 m  model_pitch=0  inertia=4000 kg*m^2  suspension_model=1  k_f=1e4 N/m  b_f=1e4 N/(m/s)  k_r=1e4 N/m  b_r=1e4 N/(m/s)  k_f_TLU=[-2000, -1000, 0, 1000, 2000] N  x_f_TLU=[-.4, -.2, 0, .2, .4] m  b_f_TLU=[-200, -100, 0, 100, 200] N  v_f_TLU=[-4, -2, 0, 2, 4] m/s  k_r_TLU=[-2000, -1000, 0, 1000, 2000] N  x_r_TLU=[-.4, -.2, 0, .2, .4] m  b_r_TLU=[-200, -100, 0, 100, 200] N  v_r_TLU=[-4, -2, 0, 2, 4] m/s  interp_method=simscape.enum.interpolation.linear  extrap_method=simscape.enum.extrapolation.linear  model_hardstop=0  upper_bound_f=.25 m  lower_bound_f=-.25 m  stop_k_f=1e6 N/m  stop_b_f=150 N/(m/s)  upper_bound_r=.25 m  lower_bound_r=-.25 m  stop_k_r=1e6 N/m  stop_b_r=150 N/(m/s)  initial_pitch=0 rad  initial_pitch_rate=0 rad/s  g=9.81 m/s^2  liftoff_warning=0  area=4 m^2  Cd=0.4  rho=1.18 kg/m^3  v_specify=on  v_priority=High  v=0 m/s  v_nominal_specify=off  v_nominal_unit=m/s  v_nominal_value=1
      settings: SourceProductName=Simscape Driveline
  Wind Velocity : fl_lib/Physical Signals/Sources/PS Constant  constant=5
  A : PMIOPort  Side=Left
  V : Outport
  wires:
  PS-Simulink Converter3/1 -> V/1  "Velocity"
  connections:
  Right Tire/RConn2 -- Left Tire/RConn2 -- Vehicle Body/LConn1
  Vehicle Body/RConn1 -- Right Tire/LConn1 -- Left Tire/LConn1
  A/RConn1 -- Right Tire/LConn2 -- Left Tire/LConn2
  PS-Simulink Converter3/LConn1 -- Vehicle Body/LConn2
  Wind Velocity/RConn1 -- Vehicle Body/LConn3
  Road Incline/RConn1 -- Vehicle Body/RConn3

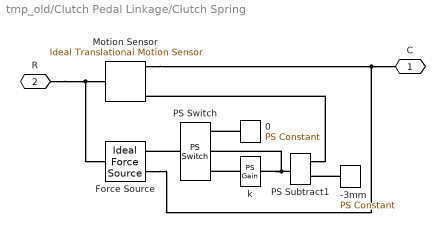
== system tmp_old/Clutch Pedal Linkage/Clutch Spring ==
  -3mm : fl_lib/Physical Signals/Sources/PS Constant  constant=-3e-3
  0 : fl_lib/Physical Signals/Sources/PS Constant  constant=0
  Force Source : fl_lib/Mechanical/Mechanical Sources/Ideal Force Source
  Motion Sensor : fl_lib/Mechanical/Mechanical Sensors/Ideal Translational Motion Sensor  offset=0 m
  PS Subtract1 : fl_lib/Physical Signals/Functions/PS Subtract
      settings: SourceProductName=Simscape
  PS Switch : fl_lib/Physical Signals/Nonlinear Operators/PS Switch  Threshold=0
      settings: SourceProductName=Simscape  SourceProductBaseCode=SS
  k : fl_lib/Physical Signals/Functions/PS Gain  gain=2000/3e-3
  C : PMIOPort  Side=Right
  R : PMIOPort  Port=2  Side=Left
  connections:
  -3mm/RConn1 -- PS Subtract1/LConn2
  Motion Sensor/RConn1 -- Force Source/RConn2 -- C/RConn1
  k/RConn1 -- PS Switch/LConn1
  PS Subtract1/LConn1 -- Motion Sensor/RConn3
  0/RConn1 -- PS Switch/LConn3
  R/RConn1 -- Motion Sensor/LConn1 -- Force Source/LConn1
  PS Subtract1/RConn1 -- PS Switch/LConn2 -- k/LConn1
  PS Switch/RConn1 -- Force Source/RConn1

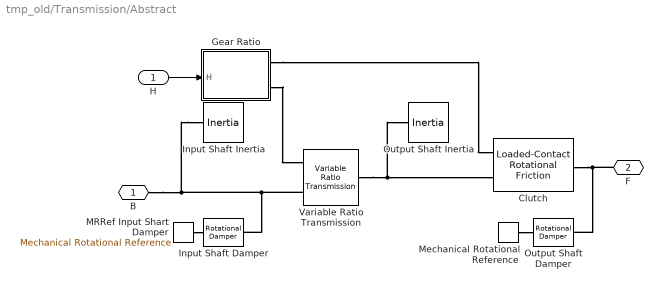
== system tmp_old/Transmission/Abstract ==
  H : Inport
  Clutch : sdl_lib/Brakes & Detents/Rotational/Loaded-Contact Rotational Friction  geometry_model=1  r_eff=300 mm  d_o=150 mm  d_i=100 mm  friction_model=1  mu_coulomb=0.46  mu_w_vector=[ 0 0.1 0.2 0.3 0.4 0.5 1 2 5 10 100 1000 ] rad/s  mu_coulomb_vector=[ 0.29 0.28 0.26 0.22 0.21 0.2 0.2 0.19 0.19 0.19 0.19 0.19 ]  mu_interp_method=1  mu_extrap_method=1  mu_static=0.5  w_tol=0.001 rad/s  force_min=100 N  mu_visc=0 N*m/(rad/s)  initial_state_locked=0  temperature_TLU=[280.0, 300.0, 320.0] K  mu_coulomb_temp_vector=[0.3, 0.28, 0.25]  mu_coulomb_matrix=[0.34, 0.32, 0.3; 0.3, 0.28, 0.25; 0.25, 0.2, 0.15]  mu_static_vector=[0.4, 0.38, 0.36]  thermal_mass=50 kJ/K  T_init=300 K
      settings: SourceProductName=Simscape Driveline  SourceProductBaseCode=LD
  Gear Ratio : Subsystem
  Input Shaft Damper : fl_lib/Mechanical/Rotational Elements/Rotational Damper  D=0.01*10 N*m/(rad/s)  w_specify=off  w_priority=High  w=0 rad/s  w_nominal_specify=off  w_nominal_unit=rad/s  w_nominal_value=1  t_specify=off  t_priority=High  t=0 N*m  t_nominal_specify=off  t_nominal_unit=N*m  t_nominal_value=1
  Input Shaft Inertia : fl_lib/Mechanical/Rotational Elements/Inertia  inertia=0.026 kg*m^2  w_specify=off  w_priority=High  w=0 rad/s  w_nominal_specify=off  w_nominal_unit=rad/s  w_nominal_value=1  t_specify=off  t_priority=High  t=0 N*m  t_nominal_specify=off  t_nominal_unit=N*m  t_nominal_value=1
  MRRef Input Shart Damper : fl_lib/Mechanical/Rotational Elements/Mechanical Rotational Reference
  Mechanical Rotational Reference : fl_lib/Mechanical/Rotational Elements/Mechanical Rotational Reference
  Output Shaft Damper : fl_lib/Mechanical/Rotational Elements/Rotational Damper  D=0.01 N*m/(rad/s)  w_specify=off  w_priority=High  w=0 rad/s  w_nominal_specify=off  w_nominal_unit=rad/s  w_nominal_value=1  t_specify=off  t_priority=High  t=0 N*m  t_nominal_specify=off  t_nominal_unit=N*m  t_nominal_value=1
  Output Shaft Inertia : fl_lib/Mechanical/Rotational Elements/Inertia  inertia=0.034 kg*m^2  w_specify=on  w_priority=High  w=0 rad/s  w_nominal_specify=off  w_nominal_unit=rad/s  w_nominal_value=1  t_specify=off  t_priority=High  t=0 N*m  t_nominal_specify=off  t_nominal_unit=N*m  t_nominal_value=1
  Variable Ratio Transmission : sdl_lib/Couplings & Drives/Variable Ratio Transmission  rotation_direction=1  kp=1e+5 N*m/rad  kv=10 N*m/(rad/s)  initial_torque=0 N*m  losses_model=1  efficiency=0.85  mu_visc=[ 0 0 ] N*m/(rad/s)  w_thr=0.01 rad/s  R_specify=off  R_priority=None  R=1  R_nominal_specify=off  R_nominal_unit=1  R_nominal_value=1
      settings: SourceProductName=Simscape Driveline  SourceProductBaseCode=LD
  B : PMIOPort  Side=Left
  F : PMIOPort  Port=2  Side=Right
  wires:
  H/1 -> Gear Ratio/1(H)
  connections:
  F/RConn1 -- Clutch/RConn1 -- Output Shaft Damper/LConn1
  MRRef Input Shart Damper/LConn1 -- Input Shaft Damper/RConn1
  Mechanical Rotational Reference/LConn1 -- Output Shaft Damper/RConn1
  Input Shaft Inertia/LConn1 -- Variable Ratio Transmission/LConn2 -- Input Shaft Damper/LConn1 -- B/RConn1
  Variable Ratio Transmission/RConn1 -- Clutch/LConn2 -- Output Shaft Inertia/LConn1
  Gear Ratio/RConn2 -- Variable Ratio Transmission/LConn1
  Gear Ratio/RConn1 -- Clutch/LConn1
